simulink model "pendulumModel"  (R2020b)
settings: Solver=ode45  StartTime=0.0  StopTime=10.0  RelTol=1e-5  AbsTol=1e-5
values from neighbouring files (symbols this model uses):
  F = 0.003    [variables.m]
  g = 9.8    [variables.m]
  I = 0.00812    [variables.m]
  L = 0.085    [variables.m]
  m = 450/1000    (= 0.45)    [variables.m]
settings Model: Creator=miastra  LastModifiedBy=miastra

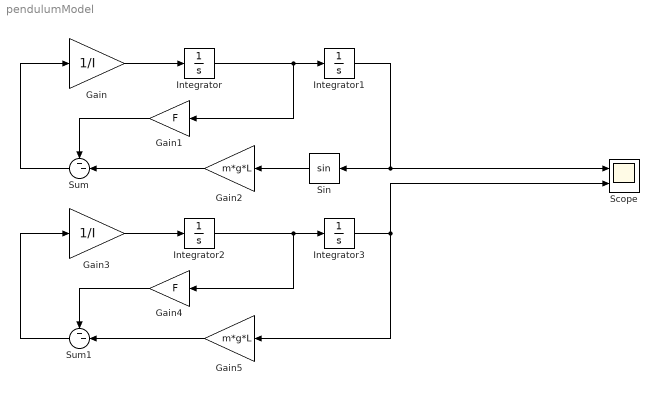
== system pendulumModel ==
  Gain : Gain  Gain=1/I
  Gain1 : Gain  Gain=F
  Gain2 : Gain  Gain=m*g*L
  Gain3 : Gain  Gain=1/I
  Gain4 : Gain  Gain=F
  Gain5 : Gain  Gain=m*g*L
  Integrator : Integrator
  Integrator1 : Integrator  InitialCondition=pi/2
  Integrator2 : Integrator
  Integrator3 : Integrator  InitialCondition=pi/2
  Scope : Scope  NumInputPorts=2
  Sin : Trigonometry
  Sum : Sum  Inputs=--|
  Sum1 : Sum  Inputs=--|
  wires:
  Integrator/1 -> Integrator1/1, Gain1/1
  Sum/1 -> Gain/1
  Gain/1 -> Integrator/1
  Gain1/1 -> Sum/1
  Integrator1/1 -> Scope/1, Sin/1
  Sin/1 -> Gain2/1
  Gain2/1 -> Sum/2
  Sum1/1 -> Gain3/1
  Gain4/1 -> Sum1/1
  Integrator2/1 -> Integrator3/1, Gain4/1
  Gain3/1 -> Integrator2/1
  Integrator3/1 -> Gain5/1, Scope/2
  Gain5/1 -> Sum1/2
